simulink model "TrayectoriaPurePursuitS_Casa"  (R2023b)
settings: Solver=FixedStepAuto  StartTime=0.0  StopTime=150  RelTol=1e-3  EnableMultiTasking=on
model workspace (MAT data in the model file):
  d = 0.19
libraries: robotalgslib x1
settings Model: ExtModeTrigDuration=2  Creator=chaya  LastModifiedBy=Usuario_UMA
settings OptimizationCC: EnhancedBackFolding=on  PassReuseOutputArgsAs=Individual arguments  ZeroExternalMemoryAtStartup=off  ZeroInternalMemoryAtStartup=off  MaxStackSize=64  OptimizeBlockOrder=speed  DifferentSizesBufferReuse=on  EfficientTunableParamExpr=on
settings DebuggingCC: ParameterTunabilityLossMsg=error
settings HardwareCC: ProdBitPerInt=16  ProdBitPerPointer=16  ProdBitPerSizeT=16  ProdBitPerPtrDiffT=16  ProdLargestAtomicFloat=None  ProdWordSize=8  ProdHWDeviceType=Atmel->AVR  UseEmbeddedCoderFeatures=off  UseSimulinkCoderFeatures=off
settings SFSimCC: MATLABDynamicMemAlloc=off
settings RTWCC: Description=Embedded Coder  SystemTargetFile=ert.tlc  HardwareBoard=Arduino Mega 2560  TemplateMakefile=ert_default_tmf  Toolchain=Arduino AVR  BuildConfiguration=Faster Runs
settings CodeAppCC: ForceParamTrailComments=on  IgnoreCustomStorageClasses=off  OperatorAnnotations=on  SimulinkDataObjDesc=on  SFDataObjDesc=on  InsertBlockDesc=on
settings ERTTargetCC: SupportContinuousTime=on  SupportNonInlinedSFcns=on  SupportVariableSizeSignals=on  ExtModeTransport=3  ExtModeStaticAlloc=on  ExtModeAutomaticAllocSize=off  ExtModeStaticAllocSize=2048  ExtModeMexFile=ext_xcp  ExtModeIntrfLevel=Level2 - Open

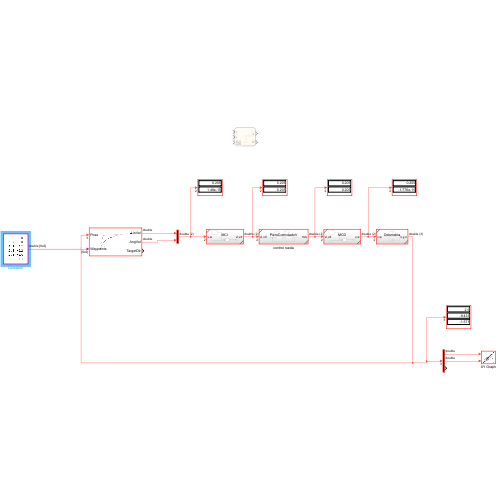
[thumbnail: Simulink's stored preview of the top-level diagram]
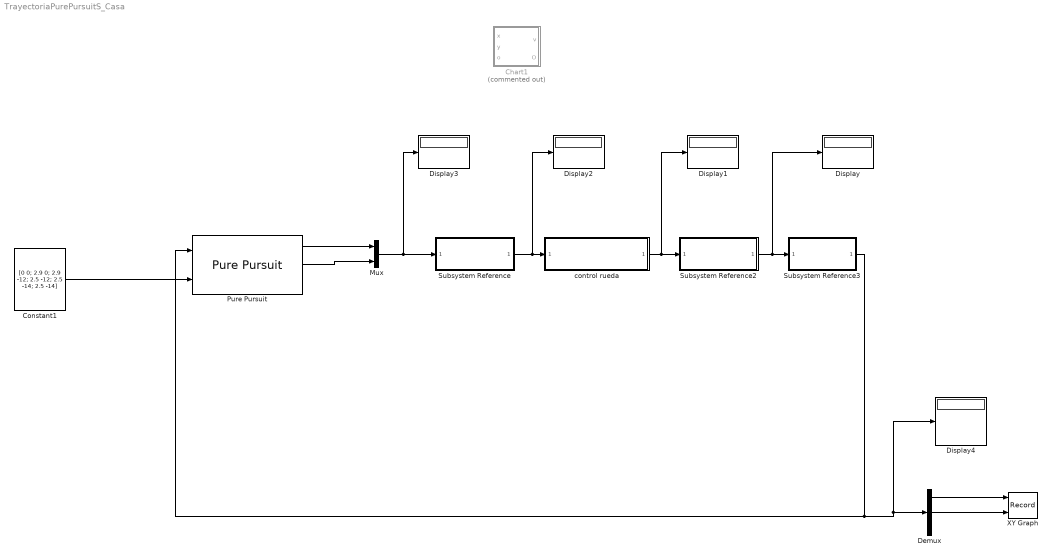
== system TrayectoriaPurePursuitS_Casa ==
  Chart1 : Stateflow chart  Commented=on  TreatAsAtomicUnit=on
  Constant1 : Constant  Value=[0 0; 2.9 0; 2.9 -12; 2.5 -12; 2.5 -14; 2.5 -14]
  Demux : Demux  Outputs=3
  Display{,1..4} (5 alike) : Display
  Mux : Mux  Inputs=2
  Pure Pursuit : robotalgslib/Pure Pursuit  DesiredLinearVelocity=0.205  MaxAngularVelocity=0.75  LookaheadDistance=0.3  TargetDirPort=on  SimulateUsing=Code generation
      settings: LibrarySourceBlock=robotmobilelib/Pure Pursuit
  Subsystem Reference : Subsystem  ReferencedSubsystem=MCI
  Subsystem Reference2 : Subsystem  ReferencedSubsystem=MCD
  Subsystem Reference3 : Subsystem  ReferencedSubsystem=Odometria
  XY Graph : Record  FileSettingsInternal="{\"entries\":[{\"content\":{\"excelSettings\":{\"content\":{},\"type\":\"Streamout.ExcelSettings\"}},\"type\":\"Streamout.FileSettingStorage\",\"uuid\":\"\"}],\"packageUris\":[\"http:\\/\\/schema.mathworks.com\\/mf0\\/streamout_blocks\\/R2020a\"],\"version\":\"1.0\"}"  Layout=[1 1]  SignalsInternal="{\"entries\":[{\"content\":{\"signals\":[{\"content\":{\"blockPath\":[],\"dimensions\":[1],\"domain\":\"\",\"lineColor\":\"#a2142f\",\"plots\":[1],\"port\":1,\"sid\":[\"\"],\"signalID\":35981,\"signalName\":\"Demux:1\"},\"type\":\"RecordBlkView.Signal\",\"uuid\":\"\"},{\"content\":{\"blockPath\":[],\"dimensions\":[1],\"domain\":\"\",\"lineColor\":\"#139fff\",\"plots\":[1],\"port\":2,\"sid\":[\"\"],\"signalID\":35985,\"signalName\":\"Demux:2\"},\"type\":\"RecordBlkView.Signal\",\"uuid\":\"\"}]},\"type\":\"RecordBlkView.InputSignals\",\"uuid\":\"\"}],\"packageUris\":[\"http:\\/\\/schema.mathworks.com\\/mf0\\/streamout_blocks\\/R2020a\"],\"version\":\"1.0\"}"  VisualizationBindings="{\"xyplotplugin\":{\"info\":[{\"series\":[{\"bindingParametersList\":[{\"parameter\":\"X-Axis\",\"signalID\":35981,\"signalName\":\"Demux:1\"},{\"parameter\":\"Y-Axis\",\"signalID\":35985,\"signalName\":\"Demux:2\"}],\"seriesID\":42193}],\"subplotID\":1}]}}"  CompatibilityTag=XY
  control rueda : Subsystem  ReferencedSubsystem=PieroControladoV
  wires:
  Subsystem Reference2/1 -> Display/1, Subsystem Reference3/1
  control rueda/1 -> Subsystem Reference2/1, Display1/1
  Subsystem Reference/1 -> control rueda/1, Display2/1
  Subsystem Reference3/1 -> Pure Pursuit/1, Display4/1, Demux/1
  Demux/1 -> XY Graph/1
  Demux/2 -> XY Graph/2
  Mux/1 -> Display3/1, Subsystem Reference/1
  Pure Pursuit/1 -> Mux/1
  Constant1/1 -> Pure Pursuit/2
  Pure Pursuit/2 -> Mux/2

== stateflow chart TrayectoriaPurePursuitS_Casa/Chart1 ==
  state Paro
    entry:
    O=pi/2;
    v=0;
  state Recto4
    entry:
    v=0.205;
    O=pi/2;
  state GiroDcha
    entry:
    v=0.1;
    O=pi;
  state Recto1
    entry:
    v=0.205;
    O=pi;
  state GiroIzq1
    entry:
    v=0.1;
    O=pi/2;
  state Recto12
    entry:
    v=0.205;
    O=pi/2;
  state Inicio
    entry:
    O=0;
    v=0;
  state Marcha
    entry:
    v=0.205;
    O=0;
  state GiroIzq
    entry:
    v=0.1;
    O=pi/2;
  Recto4 -> Paro : [y>5]
  GiroIzq1 -> Recto4 : [o<pi/2]
  GiroDcha -> Recto1 : [o>pi]
  Recto1 -> GiroIzq1 : [x<0.6]
  Recto12 -> GiroDcha : [y>1.4]
  GiroIzq -> Recto12 : [o>pi/2]
  (default) -> Inicio
  Inicio -> Marcha : [after(1,sec)]
  Marcha -> GiroIzq : [x>0.8]
  data: v output; O output; x input; y input; o input
